simulink model "PMSM_MPCC"  (R2022b)
settings: Solver=FixedStepDiscrete  StartTime=0.0  StopTime=0.5  FixedStep=1e-6  RelTol=1e-3
model workspace (MAT data in the model file):
  B = 0
  Current_Filter_On = 0
  F = 10000
  J = 5.8e-05
  Ls = 0.0005125
  Pn = 5
  Rs = 0.1445
  T = 0.0001
  T_deadband = 3e-06
  Ts = 5e-05
  Vdc = 60
  psi_f = 0.0113
  speed_ki = 1.2
  speed_kp = 0.7
undefined symbols (not defined in the file): sigbuilder_block
libraries: spsDCVoltageSourceLib x1, dspstat3 x1, spsPermanentMagnetSynchronousMachineLib x1, slpidlib x1, spsTwoLevelConverterLib x1, spspowerguiLib x1, simulink x1
(part 1 of 2)
settings Model: Creator=A  LastModifiedBy=31904
settings ModelReferenceCC: EnableRefExpFcnMdlSchedulingChecks=on

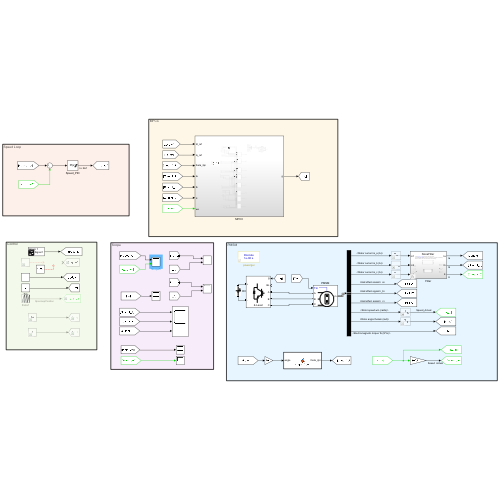
[thumbnail: Simulink's stored preview of the top-level diagram]
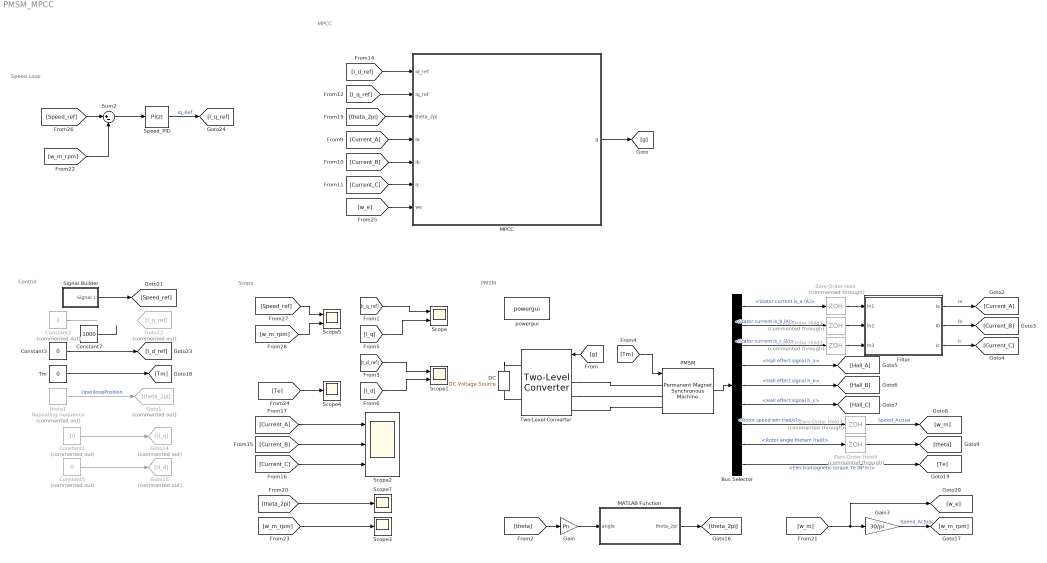
== system PMSM_MPCC ==
  note: Speed Loop
  note: Scope
  note: Control
  note: MPCC
  note: PMSM
  Bus Selector : BusSelector  OutputSignals=Stator current is_a (A),Stator current is_b (A),Stator current is_c (A),Hall effect signal h_a,Hall effect signal h_b,Hall effect signal h_c,Rotor speed wm (rad/s),Rotor angle thetam (rad),Electromagnetic torque Te (N*m)
  Constant1 : Constant  Commented=on  Value=10
  Constant2 : Constant  Commented=on  Value=2
  Constant3 : Constant  Value=0
  Constant5 : Constant  Commented=on  Value=0
  Constant7 : Constant  Value=1000
  DC : spsDCVoltageSourceLib/DC Voltage Source  Amplitude=Vdc  Measurements=None
  Filter : Subsystem  Variant=on
  Gain : Gain  Gain=Pn
  Gain3 : Gain  Gain=30/pi
  Goto1 : Goto  Commented=on  GotoTag=theta_2pi
  Goto14 : Goto  Commented=on  GotoTag=U_q
  Goto15 : Goto  Commented=on  GotoTag=U_d
  Goto22 : Goto  Commented=on  GotoTag=I_q_ref
  MATLAB Function : MATLAB Function  TreatAsAtomicUnit=on
  MPCC : Subsystem
  PMSM : spsPermanentMagnetSynchronousMachineLib/Permanent Magnet Synchronous Machine  NbPhases=3  FluxDistribution=Sinusoidal  RotorType=Round  MechanicalLoad=Torque Tm  PresetModel=No  ShowDetailedParameters=on  MeasurementBus=off  Resistance=Rs  Inductance=8.5e-3  dqInductances=[8.5e-3,8.5e-3]  La=Ls  MachineConstant=Flux linkage established by magnets (V.s)  Flux=psi_f  VoltageCst=10.248  TorqueCst=0.08475  Flat=120  Mechanical=[J B Pn 0]  PolePairs=4  InitialConditions=[0,0, 0,0]  InitialConditions5ph=[0 0 0 0 0 0]  RefAngle=Aligned with phase A axis (original Park)  IterativeDiscreteModel=Trapezoidal non iterative  TsBlock=-1  TsPowergui=0
  Scope : Scope  NumInputPorts=2
  Scope1 : Scope  NumInputPorts=2
  Scope2 : Scope  NumInputPorts=3
  Scope3 : Scope
  Scope4 : Scope
  Scope5 : Scope  NumInputPorts=2
  Scope7 : Scope
  Signal Builder : Subsystem  Tag=STV Subsys  LoadFcn=sigbuilder_block('load');  StartFcn=sigbuilder_block('start');  StopFcn=sigbuilder_block('stop');  ClipboardFcn=sigbuilder_block('clipboard');  mask(Sigbuilder block){tuvar=[0:10]}
      mask help: Simulink:masks:SigbuilderBlock_MD
      mask init:
      | if ~strcmp(get_param(bdroot(gcbh),'SimulationStatus'),'stopped') tuvar = sigbuilder_block('maskInit'); end
      settings: CopyFcn=sigbuilder_block('copy');  DeleteFcn=sigbuilder_block('delete');  ModelCloseFcn=sigbuilder_block('modelClose');  PreSaveFcn=sigbuilder_block('preSave');  PauseFcn=sigbuilder_block('pause');  ContinueFcn=sigbuilder_block('continue');  NameChangeFcn=sigbuilder_block('namechange');  OpenFcn=sigbuilder_block('open',[0 0 1152 596.4 ]);  CloseFcn=sigbuilder_block('close');
      mask Display: plot(0, 0, 100, 100,[2, 2, 32, 32, 2], [68, 8, 8, 68, 68],[32, 2], [38, 38], [32, 19, 2],[53, 60, 44], [32, 17, 17, 2],[16, 16, 31, 31]);txt = getActiveGroup(gcbh);text(2, 100, txt,'verticalAlignment', 'top');
  Speed_PID : slpidlib/PID Controller  Controller=PI  Form=Parallel  TimeDomain=Discrete-time  UseExternalTs=off  SampleTime=-1  IntegratorMethod=Forward Euler  FilterMethod=Forward Euler  ControllerParametersSource=internal  P=speed_kp  I=speed_ki  UseKiTs=off  D=0  N=100  UseFilter=on  TunerSelectOption=Transfer Function Based (PID Tuner App)  InitialConditionSource=internal  InitialConditionForIntegrator=0  InitialConditionForFilter=0  DifferentiatorICPrevScaledInput=0  ExternalReset=none  TrackingMode=off  Kt=1  LimitOutput=on  SatLimitsSource=internal  UpperSaturationLimit=Vdc  LowerSaturationLimit=-Vdc  LinearizeAsGain=on  AntiWindupMode=back-calculation  Kb=0.5  LimitIntegrator=off  UpperIntegratorSaturationLimit=inf  LowerIntegratorSaturationLimit=-inf  POutMin=[]  POutMax=[]  IOutMin=[]  IOutMax=[]  DOutMin=[]  DOutMax=[]  NOutMin=[]  NOutMax=[]  SumOutMin=[]  SumOutMax=[]  SaturationOutMin=[]  SaturationOutMax=[]  PParamMin=[]  PParamMax=[]  IParamMin=[]  IParamMax=[]  DParamMin=[]  DParamMax=[]  NParamMin=[]  NParamMax=[]  KbParamMin=[]  KbParamMax=[]  KtParamMin=[]  KtParamMax=[]  KbOutMin=[]  KbOutMax=[]  KtOutMin=[]  KtOutMax=[]  IntegratorOutMin=[]  IntegratorOutMax=[]  FilterOutMin=[]  FilterOutMax=[]  SumI1OutMin=[]  SumI1OutMax=[]  SumI2OutMin=[]  SumI2OutMax=[]  SumI3OutMin=[]  SumI3OutMax=[]  SumI4OutMin=[]  SumI4OutMax=[]  SumDOutMin=[]  SumDOutMax=[]  DifferentiatorOutMin=[]  DifferentiatorOutMax=[]  FilterDiffOutCoefMin=[]  FilterDiffOutCoefMax=[]  ReciprocalOutMin=[]  ReciprocalOutMax=[]  SumDenOutMin=[]  SumDenOutMax=[]  SumNumOutMin=[]  SumNumOutMax=[]  DivideOutMin=[]  DivideOutMax=[]  UdiffTsProdOutMin=[]  UdiffTsProdOutMax=[]  NTsProdOutMin=[]  NTsProdOutMax=[]  UintegralTsProdOutMin=[]  UintegralTsProdOutMax=[]  UngainTsProdOutMin=[]  UngainTsProdOutMax=[]  ClampingZeroOutDataTypeStr=Inherit: Inherit via back propagation  ClampingZeroOutMin=[]  ClampingZeroOutMax=[]  FilterDenConstantOutDataTypeStr=Inherit: Inherit via back propagation  FilterDenConstantOutMin=[]  FilterDenConstantOutMax=[]  PCopyOutDataTypeStr=Inherit: Inherit via back propagation  PCopyOutMin=[]  PCopyOutMax=[]  NCopyOutDataTypeStr=Inherit: Inherit via back propagation  NCopyOutMin=[]  NCopyOutMax=[]  IntegratorContinuousStateAttributes=''  IntegratorStateMustResolveToSignalObject=off  IntegratorRTWStateStorageClass=Auto  FilterContinuousStateAttributes=''  FilterStateMustResolveToSignalObject=off  FilterRTWStateStorageClass=Auto  ParallelPVariant=InternalParameters  IdealPVariant=Disabled  IVariant=InternalParameters  DVariant=Disabled  IntegratorVariant=Discrete  SatVariant=Enabled  AWVariant=BackCalculation  PCopyVariant=Disabled  TRVariant=Disabled  FdbkBlocksVariant=Forward  IdealPFdbkVariant=Disabled  SatFdbkVariant=Disabled  DerivativeFilterVariant=Disabled  NVariant=Disabled  NCopyVariant=Disabled_SignalSpec  FilterICVariant=Disabled  IntegratorICVariant=InternalICs  ExternalResetVariant=Disabled  TRSumVariant=Passthrough  SumFdbkVariant=Disabled  SumVariant=Sum_PI  TsampFilterVariant=InternalTs  TsampNgainVariant=Passthrough  TsampIntegralVariant=Passthrough  ExternalSaturationOutDataTypeStr=Inherit: Same as second input
  Sum2 : Sum  Inputs=|+-
  Tm : Constant  Value=0
  Two-Level Converter : spsTwoLevelConverterLib/Two-Level Converter  ModelType=Switching devices  Ron=1e-3  Rs=1e6  Cs=inf  Vforward=[0,0]  Ron_Diode=1e-3  Rs_Diode=1e6  Cs_Diode=inf  Vf_Diode=1e-3  Rs_CurrentSource=inf  Ron_ACsource=1e-3
  Zero-Order Hold{,1..4} (5 alike) : ZeroOrderHold  Commented=through  SampleTime=1/F
  powergui : spspowerguiLib/powergui  Priority=1  SimulationMode=Discrete  SampleTime=1e-6  frequency=60  Iterations=50  frequencyindice=0  Pbase=100e6  ErrMax=1e-4  UnitsV=kV  UnitsW=MW  buscounter=0  FunctionMessages=off  echomessages=off  EnableUseOfTLC=off  CurrentSourceSwitches=off  DisableSnubberDevices=off  DisableRonSwitches=off  DisableVfSwitches=off  DisplayEquations=off  AutomaticDiscreteSolvers=off  SolverType=Tustin/Backward Euler (TBE)  Interpol=off  ExternalGateDelay=off  methode=off  Ts=100  x0status=blocks  SPID=on  SwTol=0  HookPort=off  NonlinearTolerance=1e-4  nMaxIteration=100  ContinueOnMaxIteration=off  RestoreLinks=warning  ResistiveCurrentMeasurement=off  Frange=[0:2:500]  Ylog=off  Xlog=on  ShowGrid=off  save=off  variable=ZData  structure=0  ZoomFFT=off  StartTime=0.0  cycles=1  DisplayStyle=1  fundamental=60  FreqAxis=off  MaxFrequency=1000  frequencyindicesteady=1  RmsSteady=1  display=off
  theta1 : simulink/Sources/Repeating Sequence  Commented=on  rep_seq_t=[0 0.1]  rep_seq_y=[0 2*pi]
  wires:
  [theta_2pi] -> MPCC/3(theta_2pi)
  [Current_A] -> MPCC/4(Ia)
  [Current_C] -> MPCC/6(Ic)
  [Current_B] -> MPCC/5(Ib)
  Zero-Order Hold4/1 -> [theta]
  Bus Selector/1 -> Zero-Order Hold/1  "<Stator current is_a (A)>"
  Zero-Order Hold/1 -> Filter/1(ln1)
  Zero-Order Hold1/1 -> Filter/2(ln2)
  Bus Selector/4 -> [Hall_A]  "<Hall effect signal h_a>"
  [theta] -> Gain/1
  Bus Selector/2 -> Zero-Order Hold1/1  "<Stator current is_b (A)>"
  [g] -> Two-Level Converter/1
  Bus Selector/3 -> Zero-Order Hold2/1  "<Stator current is_c (A)>"
  [Tm] -> PMSM/1
  Zero-Order Hold3/1 -> [w_m]  "Speed_Actual"
  Bus Selector/8 -> Zero-Order Hold4/1  "<Rotor angle thetam (rad)>"
  MATLAB Function/1(theta_2pi) -> [theta_2pi]
  Bus Selector/7 -> Zero-Order Hold3/1  "<Rotor speed wm (rad/s)>"
  PMSM/1 -> Bus Selector/1
  Bus Selector/5 -> [Hall_B]  "<Hall effect signal h_b>"
  Zero-Order Hold2/1 -> Filter/3(ln3)
  Bus Selector/6 -> [Hall_C]  "<Hall effect signal h_c>"
  Constant3/1 -> [I_d_ref]
  Constant2/1 -> ?
  [I_q_ref] -> Scope/1
  [I_q] -> Scope/2
  [I_d_ref] -> Scope1/1
  [I_d] -> Scope1/2
  [I_q_ref] -> MPCC/2(Iq_ref)
  [Current_C] -> Scope2/3
  [Current_B] -> Scope2/2
  [Current_A] -> Scope2/1
  [theta_2pi] -> Scope7/1
  Filter/1(Ia) -> [Current_A]  "Ia"
  Filter/2(Ib) -> [Current_B]  "Ib"
  Filter/3(Ic) -> [Current_C]  "Ic"
  MPCC/1(g) -> [g]
  theta1/1 -> Goto1/1  "OpenloopPosition"
  Constant5/1 -> Goto15/1
  Constant1/1 -> Goto14/1
  [w_m] -> [w_e], Gain3/1
  Gain3/1 -> [w_m_rpm]  "Speed_Actual"
  [w_m_rpm] -> Scope3/1
  Gain/1 -> MATLAB Function/1(angle)
  Tm/1 -> [Tm]
  Bus Selector/9 -> [Te]  "<Electromagnetic torque Te (N*m)>"
  [Te] -> Scope4/1
  [w_e] -> MPCC/7(we)
  Constant7/1 -> ?
  Sum2/1 -> Speed_PID/1
  [w_m_rpm] -> Sum2/2
  [Speed_ref] -> Sum2/1
  Speed_PID/1 -> [I_q_ref]  "Iq_Ref"
  [Speed_ref] -> Scope5/1
  [w_m_rpm] -> Scope5/2
  Signal Builder/1(Signal 1) -> [Speed_ref]
  [I_d_ref] -> MPCC/1(Id_ref)
  connections:
  DC/LConn1 -- Two-Level Converter/RConn2
  DC/RConn1 -- Two-Level Converter/RConn1
  PMSM/LConn3 -- Two-Level Converter/LConn3
  Two-Level Converter/LConn1 -- PMSM/LConn1
  Two-Level Converter/LConn2 -- PMSM/LConn2

== system PMSM_MPCC/Filter ==
  note: 1) Add Subsystem or Model blocks as valid variant choices.
      | 2) You cannot connect blocks at this level. At simulation, connectivity is automatically
      | determined, based on the active variant and port name matching.
  ln1 : Inport
  ln2 : Inport  Port=2
  ln3 : Inport  Port=3
  LowpassFilter : Subsystem  VariantControl=Current_Filter_On==1
  NoneFilter : Subsystem  VariantControl=Current_Filter_On==0
  Ia : Outport
  Ib : Outport  Port=2
  Ic : Outport  Port=3

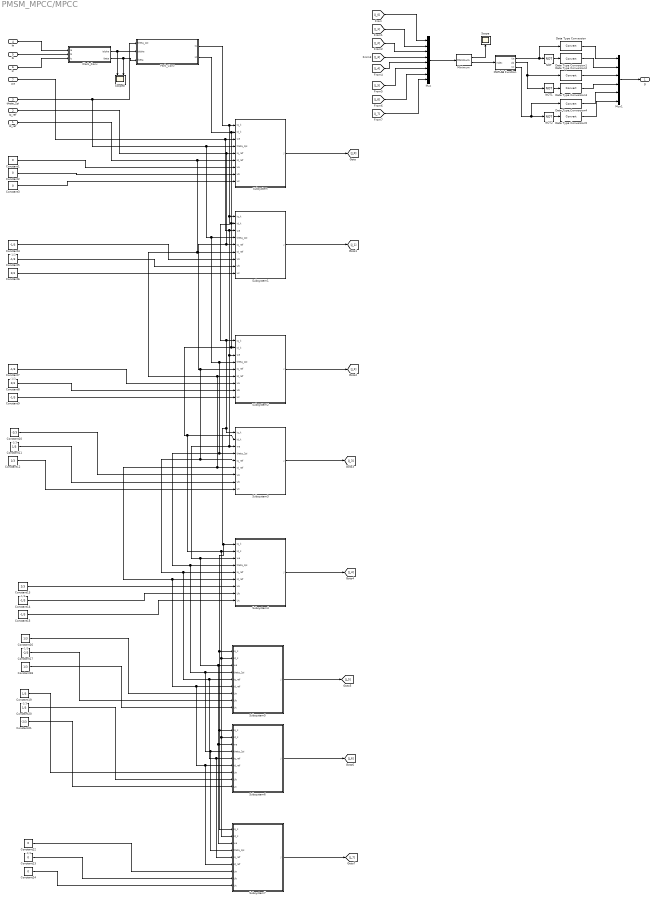
== system PMSM_MPCC/MPCC ==
  note: -1/3
  note: -1/3
  note: -1/3
  note: -1/3
  note: -1/3
  note: -1/3
  note: -1/3
  Id_ref : Inport
  Iq_ref : Inport  Port=2
  theta_2pi : Inport  Port=3
  Ia : Inport  Port=4
  Ib : Inport  Port=5
  Ic : Inport  Port=6
  we : Inport  Port=7
  Clark_Conv : Subsystem
  Constant{1..3,22..24} (6 alike) : Constant  Value=0
  Constant10 : Constant  Value=-2/3
  Constant{11..12,16,18..20} (6 alike) : Constant  Value=1/3
  Constant13 : Constant  Value=2/3
  Constant{4..5,7,9,14..15} (6 alike) : Constant  Value=-1/3
  Constant17 : Constant  Value=-2/3
  Constant21 : Constant  Value=-2/3
  Constant6 : Constant  Value=2/3
  Constant8 : Constant  Value=2/3
  Data Type Conversion{,1..5} (6 alike) : DataTypeConversion  SaturateOnIntegerOverflow=off  RndMeth=Floor
  MATLAB Function : MATLAB Function  TreatAsAtomicUnit=on
  Minimum : dspstat3/Minimum  operation=minimum  fcn=Value and Index  indexBase=Zero  operateOver=Entire input  Dimension=1  InputProcessing=Columns as channels (frame based)  reset=None  roiEnable=off  roiType=Rectangles  roiPortion=Entire ROI  roiOutput=Individual statistics for each ROI  roiFlag=off  roundingMode=Floor  overflowMode=off
      settings: LibrarySourceBlock=dsphdlsupportstat/Minimum
  Mux : Mux  Inputs=8
  Mux1 : Mux  Inputs=6
  NOT : Logic  Operator=NOT  IconShape=distinctive  AllPortsSameDT=off  OutDataTypeStr=boolean
  NOT1 : Logic  Operator=NOT  IconShape=distinctive  AllPortsSameDT=off  OutDataTypeStr=boolean
  NOT2 : Logic  Operator=NOT  IconShape=distinctive  AllPortsSameDT=off  OutDataTypeStr=boolean
  Park_Conv : Subsystem
  Scope : Scope
  Scope8 : Scope  NumInputPorts=2
  Subsystem : Subsystem
  Subsystem1 : Subsystem
  Subsystem2 : Subsystem
  Subsystem3 : Subsystem
  Subsystem4 : Subsystem
  Subsystem5 : Subsystem
  Subsystem6 : Subsystem
  Subsystem7 : Subsystem
  g : Outport
  wires:
  Clark_Conv/1(Ialpha) -> Park_Conv/2(Ialpha), Scope8/1
  theta_2pi/1 -> Park_Conv/1(theta_2pi), Subsystem/4(theta_2pi), Subsystem3/4(theta_2pi), Subsystem7/4(theta_2pi), Subsystem6/4(theta_2pi), Subsystem5/4(theta_2pi), Subsystem4/4(theta_2pi), Subsystem2/4(theta_2pi), Subsystem1/4(theta_2pi)
  Clark_Conv/2(Ibeta) -> Park_Conv/3(Ibeta), Scope8/2
  Mux1/1 -> g/1
  Ic/1 -> Clark_Conv/3(Ic)
  Ib/1 -> Clark_Conv/2(Ib)
  Ia/1 -> Clark_Conv/1(Ia)
  Constant22/1 -> Subsystem7/7(Ua)
  Constant24/1 -> Subsystem7/9(Uc)
  Constant12/1 -> Subsystem3/9(Uc)
  Constant19/1 -> Subsystem6/7(Ua)
  Constant20/1 -> Subsystem6/8(Ub)
  Constant11/1 -> Subsystem3/8(Ub)
  Constant10/1 -> Subsystem3/7(Ua)
  Constant7/1 -> Subsystem2/7(Ua)
  Constant8/1 -> Subsystem2/8(Ub)
  Constant9/1 -> Subsystem2/9(Uc)
  Constant4/1 -> Subsystem1/7(Ua)
  Constant5/1 -> Subsystem1/8(Ub)
  Constant6/1 -> Subsystem1/9(Uc)
  Constant17/1 -> Subsystem5/8(Ub)
  Constant23/1 -> Subsystem7/8(Ub)
  Constant16/1 -> Subsystem5/7(Ua)
  Constant15/1 -> Subsystem4/9(Uc)
  Constant18/1 -> Subsystem5/9(Uc)
  Constant21/1 -> Subsystem6/9(Uc)
  Constant14/1 -> Subsystem4/8(Ub)
  Constant13/1 -> Subsystem4/7(Ua)
  Park_Conv/1(Iq) -> Subsystem7/1(iq_k), Subsystem6/1(iq_k), Subsystem5/1(iq_k), Subsystem4/1(iq_k), Subsystem3/1(iq_k), Subsystem2/1(iq_k), Subsystem1/1(iq_k), Subsystem/1(iq_k)
  Park_Conv/2(Id) -> Subsystem7/2(id_k), Subsystem6/2(id_k), Subsystem5/2(id_k), Subsystem4/2(id_k), Subsystem3/2(id_k), Subsystem2/2(id_k), Subsystem1/2(id_k), Subsystem/2(id_k)
  we/1 -> Subsystem3/3(we), Subsystem7/3(we), Subsystem6/3(we), Subsystem5/3(we), Subsystem4/3(we), Subsystem2/3(we), Subsystem1/3(we), Subsystem/3(we)
  Iq_ref/1 -> Subsystem1/5(Iq_ref), Subsystem3/5(Iq_ref), Subsystem7/5(Iq_ref), Subsystem6/5(Iq_ref), Subsystem5/5(Iq_ref), Subsystem4/5(Iq_ref), Subsystem2/5(Iq_ref), Subsystem/5(Iq_ref)
  Id_ref/1 -> Subsystem1/6(Id_ref), Subsystem3/6(Id_ref), Subsystem7/6(Id_ref), Subsystem6/6(Id_ref), Subsystem5/6(Id_ref), Subsystem4/6(Id_ref), Subsystem2/6(Id_ref), Subsystem/6(Id_ref)
  Constant1/1 -> Subsystem/7(Ua)
  Constant2/1 -> Subsystem/8(Ub)
  Constant3/1 -> Subsystem/9(Uc)
  Subsystem/1(J) -> [J_0]
  Subsystem1/1(J) -> [J_1]
  Subsystem2/1(J) -> [J_2]
  Subsystem3/1(J) -> [J_3]
  Subsystem4/1(J) -> [J_4]
  Subsystem5/1(J) -> [J_5]
  Subsystem6/1(J) -> [J_6]
  Subsystem7/1(J) -> [J_7]
  [J_0] -> Mux/1
  [J_1] -> Mux/2
  [J_2] -> Mux/3
  [J_3] -> Mux/4
  [J_4] -> Mux/5
  [J_5] -> Mux/6
  [J_6] -> Mux/7
  [J_7] -> Mux/8
  Mux/1 -> Minimum/1
  Minimum/1 -> Scope/1
  Minimum/2 -> MATLAB Function/1(index)
  MATLAB Function/1(Ua) -> Data Type Conversion/1, NOT/1
  NOT/1 -> Data Type Conversion1/1
  Data Type Conversion/1 -> Mux1/1
  Data Type Conversion1/1 -> Mux1/2
  Data Type Conversion2/1 -> Mux1/3
  Data Type Conversion3/1 -> Mux1/4
  NOT1/1 -> Data Type Conversion3/1
  MATLAB Function/2(Ub) -> Data Type Conversion2/1, NOT1/1
  Data Type Conversion4/1 -> Mux1/5
  Data Type Conversion5/1 -> Mux1/6
  NOT2/1 -> Data Type Conversion5/1
  MATLAB Function/3(Uc) -> Data Type Conversion4/1, NOT2/1

== system PMSM_MPCC/Signal Builder ==
  Demux : Demux  Tag=STV Demux  Outputs=1
      settings: DisplayOption=none
  FromWs : FromWorkspace  Tag=STV FromWs  VariableName=tuvar
      SigBuilderData=|
      | common.afterFinalStr = 'Extrapolate'
      | common.sampleTime = 0
      | dataSet.timeRange = [0 1]
      | dataSet.name = 'Group 1'
      | sbobj.Groups.Name = 'Group 1'
      | sbobj.Groups.Signals.Name = 'Signal 1'
      | sbobj.Groups.Signals.XData = [0 0.2 0.2 0.3 0.3 0.5 0.5 0.6 0.6 0.8 0.8 0.9 0.9 1]
      | sbobj.Groups.Signals.YData = [1000 1000 3000 3000 5000 5000 4000 4000 2000 2000 1000 1000 0 0]
      | sbobj.Groups.TimeRange = [0 1]
  Signal 1 : Outport  Tag=STV Outport
  wires:
  Demux/1 -> Signal 1/1
  FromWs/1 -> Demux/1

== system PMSM_MPCC/Filter/LowpassFilter ==
  ln1 : Inport
  ln2 : Inport  Port=2
  ln3 : Inport  Port=3
  Lowpass filter1 : Subsystem
  Lowpass filter2 : Subsystem
  Lowpass filter3 : Subsystem
  a : Constant  Value=0.001
  Ia : Outport
  Ib : Outport  Port=2
  Ic : Outport  Port=3
  wires:
  ln2/1 -> Lowpass filter2/2(u(t))
  a/1 -> Lowpass filter3/1(K), Lowpass filter2/1(K), Lowpass filter1/1(K)
  ln1/1 -> Lowpass filter1/2(u(t))
  Lowpass filter1/1(Ia) -> Ia/1
  Lowpass filter2/1(Ib) -> Ib/1
  Lowpass filter3/1(Ic) -> Ic/1
  ln3/1 -> Lowpass filter3/2(u(t))

== system PMSM_MPCC/Filter/NoneFilter ==
  ln1 : Inport
  ln2 : Inport  Port=2
  ln3 : Inport  Port=3
  Ia : Outport
  Ib : Outport  Port=2
  Ic : Outport  Port=3
  wires:
  ln1/1 -> Ia/1
  ln2/1 -> Ib/1
  ln3/1 -> Ic/1

== system PMSM_MPCC/MPCC/Clark_Conv ==
  Ia : Inport
  Ib : Inport  Port=2
  Ic : Inport  Port=3
  Add : Sum  Inputs=+-  OutDataTypeStr=double
  Gain : Gain  Gain=sqrt(3)  ParamDataTypeStr=double
  Gain2 : Gain  Gain=0.5
  Gain3 : Gain  Gain=0.5
  Subtract : Sum  Inputs=+--  OutDataTypeStr=double
  Ialpha : Outport
  Ibeta : Outport  Port=2
  wires:
  Ia/1 -> Subtract/1
  Ib/1 -> Gain2/1
  Add/1 -> Gain/1
  Gain/1 -> Ibeta/1
  Ic/1 -> Gain3/1
  Gain2/1 -> Subtract/2, Add/1
  Gain3/1 -> Subtract/3, Add/2
  Subtract/1 -> Ialpha/1

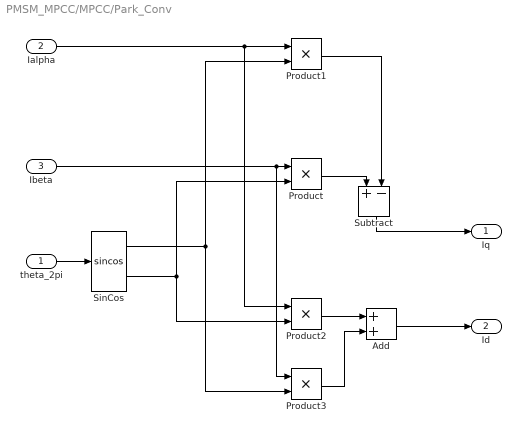
== system PMSM_MPCC/MPCC/Park_Conv ==
  theta_2pi : Inport
  Ialpha : Inport  Port=2
  Ibeta : Inport  Port=3
  Add : Sum
  Product{,1..3} (4 alike) : Product
  SinCos : Trigonometry  Operator=sincos
  Subtract : Sum  Inputs=+-
  Iq : Outport
  Id : Outport  Port=2
  wires:
  Ialpha/1 -> Product1/1, Product2/1
  Ibeta/1 -> Product3/1, Product/1
  theta_2pi/1 -> SinCos/1
  SinCos/2 -> Product2/2, Product/2
  SinCos/1 -> Product3/2, Product1/2
  Product1/1 -> Subtract/2
  Subtract/1 -> Iq/1
  Product/1 -> Subtract/1
  Product2/1 -> Add/1
  Product3/1 -> Add/2
  Add/1 -> Id/1

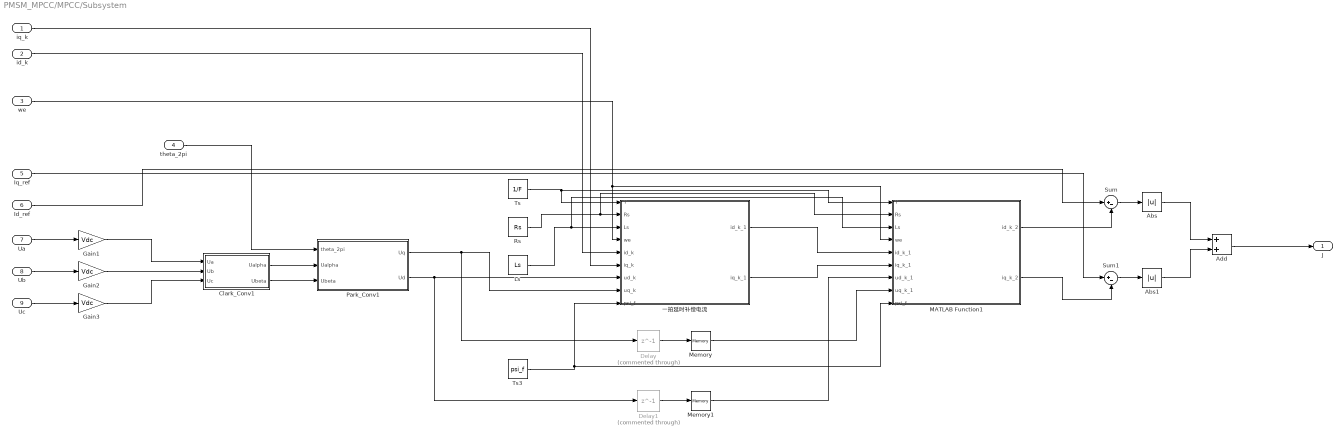
== system PMSM_MPCC/MPCC/Subsystem ==
  iq_k : Inport
  id_k : Inport  Port=2
  we : Inport  Port=3
  theta_2pi : Inport  Port=4
  Iq_ref : Inport  Port=5
  Id_ref : Inport  Port=6
  Ua : Inport  Port=7
  Ub : Inport  Port=8
  Uc : Inport  Port=9
  Abs : Abs  SaturateOnIntegerOverflow=off
  Abs1 : Abs  SaturateOnIntegerOverflow=off
  Add : Sum
  Clark_Conv1 : Subsystem
  Delay : Delay  Commented=through  DelayLength=1
  Delay1 : Delay  Commented=through  DelayLength=1
  Gain1 : Gain  Gain=Vdc
  Gain2 : Gain  Gain=Vdc
  Gain3 : Gain  Gain=Vdc
  Ls : Constant  Value=Ls
  MATLAB Function1 : MATLAB Function  TreatAsAtomicUnit=on
  Memory : Memory
  Memory1 : Memory
  Park_Conv1 : Subsystem
  Rs : Constant  Value=Rs
  Sum : Sum  Inputs=|+-
  Sum1 : Sum  Inputs=|+-
  Ts : Constant  Value=1/F
  Ts3 : Constant  Value=psi_f
  一拍延时补偿电流 : MATLAB Function  TreatAsAtomicUnit=on
  J : Outport
  wires:
  Park_Conv1/1(Uq) -> Delay/1, 一拍延时补偿电流/8(uq_k)
  MATLAB Function1/2(iq_k_2) -> Sum1/2
  Iq_ref/1 -> Sum1/1
  theta_2pi/1 -> Park_Conv1/1(theta_2pi)
  Sum/1 -> Abs/1
  一拍延时补偿电流/2(iq_k_1) -> MATLAB Function1/6(iq_k_1)
  Rs/1 -> MATLAB Function1/2(Rs), 一拍延时补偿电流/2(Rs)
  Delay/1 -> Memory/1
  MATLAB Function1/1(id_k_2) -> Sum/2
  Add/1 -> J/1
  Ts/1 -> MATLAB Function1/1(T), 一拍延时补偿电流/1(T)
  一拍延时补偿电流/1(id_k_1) -> MATLAB Function1/5(id_k_1)
  Park_Conv1/2(Ud) -> Delay1/1, 一拍延时补偿电流/7(ud_k)
  Gain1/1 -> Clark_Conv1/1(Ua)
  Gain2/1 -> Clark_Conv1/2(Ub)
  Ls/1 -> MATLAB Function1/3(Ls), 一拍延时补偿电流/3(Ls)
  Clark_Conv1/2(Ubeta) -> Park_Conv1/3(Ubeta)
  Sum1/1 -> Abs1/1
  Gain3/1 -> Clark_Conv1/3(Uc)
  Abs/1 -> Add/1
  Id_ref/1 -> Sum/1
  we/1 -> 一拍延时补偿电流/4(we), MATLAB Function1/4(we)
  Delay1/1 -> Memory1/1
  Ua/1 -> Gain1/1
  Ts3/1 -> MATLAB Function1/9(psi_f), 一拍延时补偿电流/9(psi_f)
  Abs1/1 -> Add/2
  Clark_Conv1/1(Ualpha) -> Park_Conv1/2(Ualpha)
  id_k/1 -> 一拍延时补偿电流/5(id_k)
  iq_k/1 -> 一拍延时补偿电流/6(iq_k)
  Ub/1 -> Gain2/1
  Uc/1 -> Gain3/1
  Memory/1 -> MATLAB Function1/8(uq_k_1)
  Memory1/1 -> MATLAB Function1/7(ud_k_1)

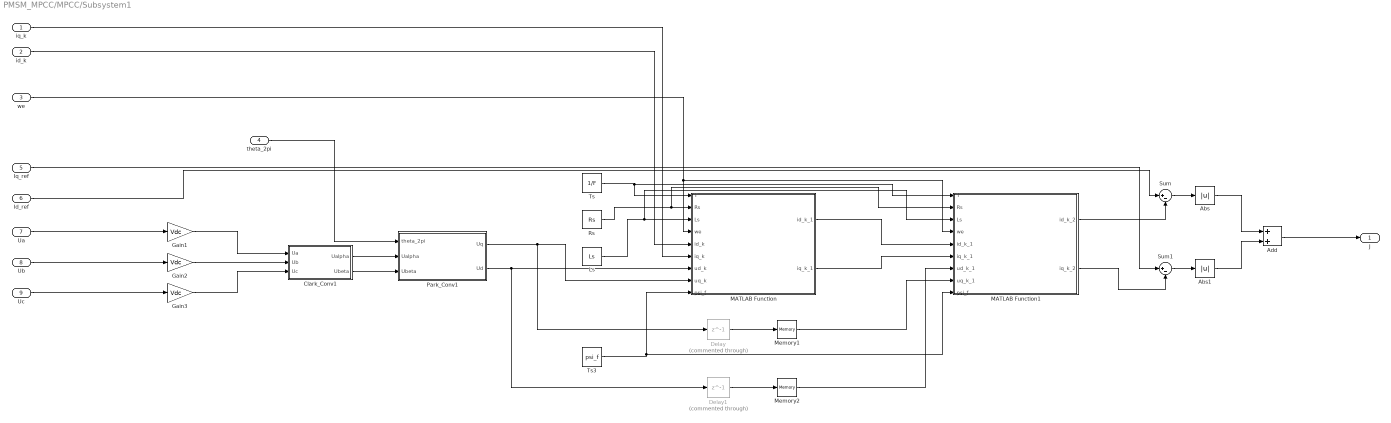
== system PMSM_MPCC/MPCC/Subsystem1 ==
  iq_k : Inport
  id_k : Inport  Port=2
  we : Inport  Port=3
  theta_2pi : Inport  Port=4
  Iq_ref : Inport  Port=5
  Id_ref : Inport  Port=6
  Ua : Inport  Port=7
  Ub : Inport  Port=8
  Uc : Inport  Port=9
  Abs : Abs  SaturateOnIntegerOverflow=off
  Abs1 : Abs  SaturateOnIntegerOverflow=off
  Add : Sum
  Clark_Conv1 : Subsystem
  Delay : Delay  Commented=through  DelayLength=1
  Delay1 : Delay  Commented=through  DelayLength=1
  Gain1 : Gain  Gain=Vdc
  Gain2 : Gain  Gain=Vdc
  Gain3 : Gain  Gain=Vdc
  Ls : Constant  Value=Ls
  MATLAB Function : MATLAB Function  TreatAsAtomicUnit=on
  MATLAB Function1 : MATLAB Function  TreatAsAtomicUnit=on
  Memory1 : Memory
  Memory2 : Memory
  Park_Conv1 : Subsystem
  Rs : Constant  Value=Rs
  Sum : Sum  Inputs=|+-
  Sum1 : Sum  Inputs=|+-
  Ts : Constant  Value=1/F
  Ts3 : Constant  Value=psi_f
  J : Outport
  wires:
  Uc/1 -> Gain3/1
  Ub/1 -> Gain2/1
  iq_k/1 -> MATLAB Function/6(iq_k)
  id_k/1 -> MATLAB Function/5(id_k)
  Clark_Conv1/1(Ualpha) -> Park_Conv1/2(Ualpha)
  Abs1/1 -> Add/2
  Ts3/1 -> MATLAB Function/9(psi_f), MATLAB Function1/9(psi_f)
  Ua/1 -> Gain1/1
  Delay1/1 -> Memory2/1
  we/1 -> MATLAB Function1/4(we), MATLAB Function/4(we)
  Id_ref/1 -> Sum/1
  Abs/1 -> Add/1
  Gain3/1 -> Clark_Conv1/3(Uc)
  Sum1/1 -> Abs1/1
  Clark_Conv1/2(Ubeta) -> Park_Conv1/3(Ubeta)
  Ls/1 -> MATLAB Function/3(Ls), MATLAB Function1/3(Ls)
  Gain2/1 -> Clark_Conv1/2(Ub)
  Gain1/1 -> Clark_Conv1/1(Ua)
  Park_Conv1/2(Ud) -> MATLAB Function/7(ud_k), Delay1/1
  MATLAB Function/1(id_k_1) -> MATLAB Function1/5(id_k_1)
  Ts/1 -> MATLAB Function/1(T), MATLAB Function1/1(T)
  Add/1 -> J/1
  MATLAB Function1/1(id_k_2) -> Sum/2
  Delay/1 -> Memory1/1
  Rs/1 -> MATLAB Function/2(Rs), MATLAB Function1/2(Rs)
  MATLAB Function/2(iq_k_1) -> MATLAB Function1/6(iq_k_1)
  Sum/1 -> Abs/1
  theta_2pi/1 -> Park_Conv1/1(theta_2pi)
  Iq_ref/1 -> Sum1/1
  MATLAB Function1/2(iq_k_2) -> Sum1/2
  Park_Conv1/1(Uq) -> MATLAB Function/8(uq_k), Delay/1
  Memory1/1 -> MATLAB Function1/8(uq_k_1)
  Memory2/1 -> MATLAB Function1/7(ud_k_1)

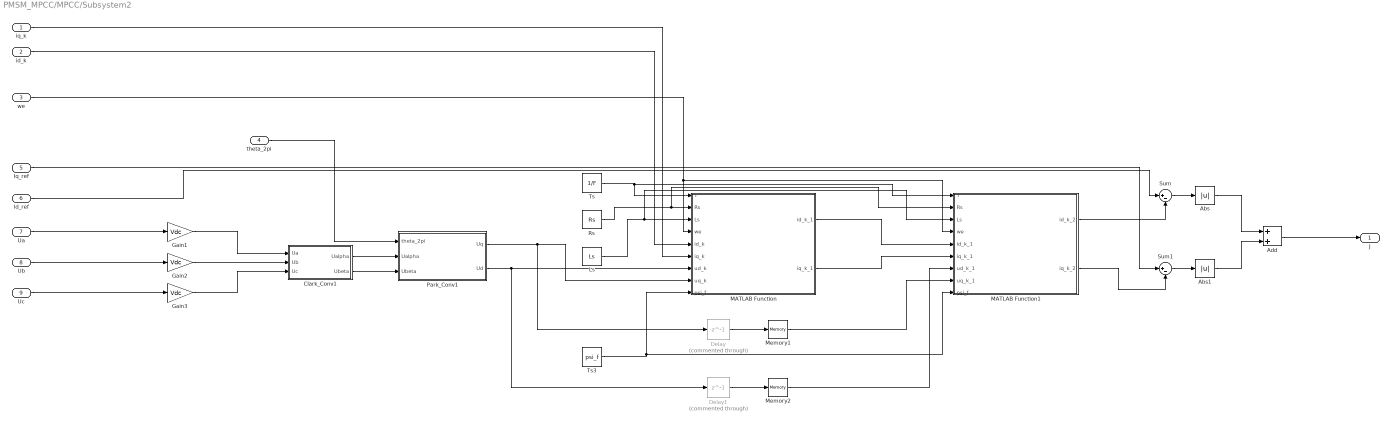
== system PMSM_MPCC/MPCC/Subsystem2 ==
  iq_k : Inport
  id_k : Inport  Port=2
  we : Inport  Port=3
  theta_2pi : Inport  Port=4
  Iq_ref : Inport  Port=5
  Id_ref : Inport  Port=6
  Ua : Inport  Port=7
  Ub : Inport  Port=8
  Uc : Inport  Port=9
  Abs : Abs  SaturateOnIntegerOverflow=off
  Abs1 : Abs  SaturateOnIntegerOverflow=off
  Add : Sum
  Clark_Conv1 : Subsystem
  Delay : Delay  Commented=through  DelayLength=1
  Delay1 : Delay  Commented=through  DelayLength=1
  Gain1 : Gain  Gain=Vdc
  Gain2 : Gain  Gain=Vdc
  Gain3 : Gain  Gain=Vdc
  Ls : Constant  Value=Ls
  MATLAB Function : MATLAB Function  TreatAsAtomicUnit=on
  MATLAB Function1 : MATLAB Function  TreatAsAtomicUnit=on
  Memory1 : Memory
  Memory2 : Memory
  Park_Conv1 : Subsystem
  Rs : Constant  Value=Rs
  Sum : Sum  Inputs=|+-
  Sum1 : Sum  Inputs=|+-
  Ts : Constant  Value=1/F
  Ts3 : Constant  Value=psi_f
  J : Outport
  wires:
  Uc/1 -> Gain3/1
  Ub/1 -> Gain2/1
  iq_k/1 -> MATLAB Function/6(iq_k)
  id_k/1 -> MATLAB Function/5(id_k)
  Clark_Conv1/1(Ualpha) -> Park_Conv1/2(Ualpha)
  Abs1/1 -> Add/2
  Ts3/1 -> MATLAB Function/9(psi_f), MATLAB Function1/9(psi_f)
  Ua/1 -> Gain1/1
  Delay1/1 -> Memory2/1
  we/1 -> MATLAB Function1/4(we), MATLAB Function/4(we)
  Id_ref/1 -> Sum/1
  Abs/1 -> Add/1
  Gain3/1 -> Clark_Conv1/3(Uc)
  Sum1/1 -> Abs1/1
  Clark_Conv1/2(Ubeta) -> Park_Conv1/3(Ubeta)
  Ls/1 -> MATLAB Function/3(Ls), MATLAB Function1/3(Ls)
  Gain2/1 -> Clark_Conv1/2(Ub)
  Gain1/1 -> Clark_Conv1/1(Ua)
  Park_Conv1/2(Ud) -> MATLAB Function/7(ud_k), Delay1/1
  MATLAB Function/1(id_k_1) -> MATLAB Function1/5(id_k_1)
  Ts/1 -> MATLAB Function/1(T), MATLAB Function1/1(T)
  Add/1 -> J/1
  MATLAB Function1/1(id_k_2) -> Sum/2
  Delay/1 -> Memory1/1
  Rs/1 -> MATLAB Function/2(Rs), MATLAB Function1/2(Rs)
  MATLAB Function/2(iq_k_1) -> MATLAB Function1/6(iq_k_1)
  Sum/1 -> Abs/1
  theta_2pi/1 -> Park_Conv1/1(theta_2pi)
  Iq_ref/1 -> Sum1/1
  MATLAB Function1/2(iq_k_2) -> Sum1/2
  Park_Conv1/1(Uq) -> MATLAB Function/8(uq_k), Delay/1
  Memory1/1 -> MATLAB Function1/8(uq_k_1)
  Memory2/1 -> MATLAB Function1/7(ud_k_1)

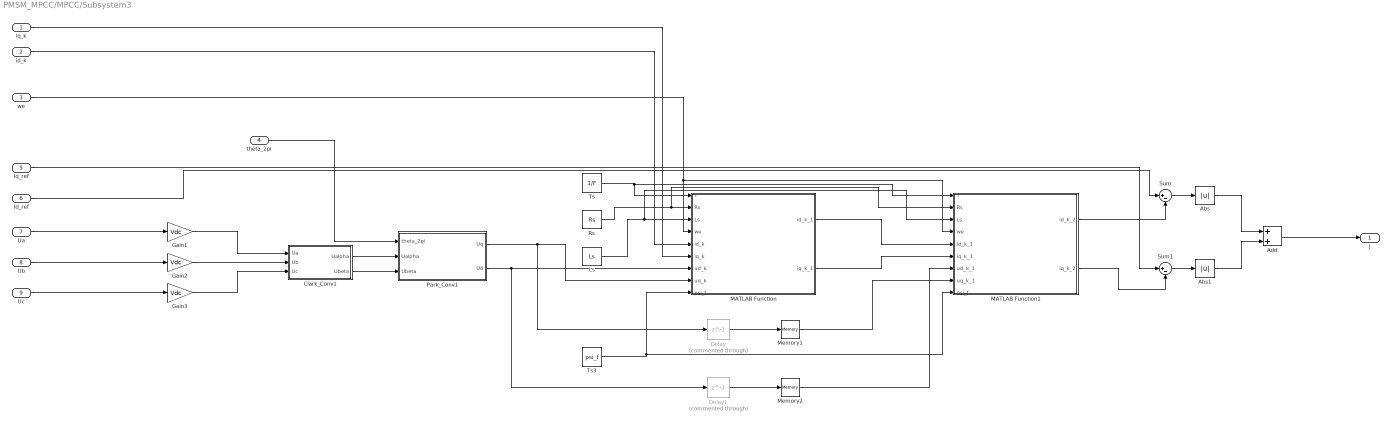
== system PMSM_MPCC/MPCC/Subsystem3 ==
  iq_k : Inport
  id_k : Inport  Port=2
  we : Inport  Port=3
  theta_2pi : Inport  Port=4
  Iq_ref : Inport  Port=5
  Id_ref : Inport  Port=6
  Ua : Inport  Port=7
  Ub : Inport  Port=8
  Uc : Inport  Port=9
  Abs : Abs  SaturateOnIntegerOverflow=off
  Abs1 : Abs  SaturateOnIntegerOverflow=off
  Add : Sum
  Clark_Conv1 : Subsystem
  Delay : Delay  Commented=through  DelayLength=1
  Delay1 : Delay  Commented=through  DelayLength=1
  Gain1 : Gain  Gain=Vdc
  Gain2 : Gain  Gain=Vdc
  Gain3 : Gain  Gain=Vdc
  Ls : Constant  Value=Ls
  MATLAB Function : MATLAB Function  TreatAsAtomicUnit=on
  MATLAB Function1 : MATLAB Function  TreatAsAtomicUnit=on
  Memory1 : Memory
  Memory2 : Memory
  Park_Conv1 : Subsystem
  Rs : Constant  Value=Rs
  Sum : Sum  Inputs=|+-
  Sum1 : Sum  Inputs=|+-
  Ts : Constant  Value=1/F
  Ts3 : Constant  Value=psi_f
  J : Outport
  wires:
  Uc/1 -> Gain3/1
  Ub/1 -> Gain2/1
  iq_k/1 -> MATLAB Function/6(iq_k)
  id_k/1 -> MATLAB Function/5(id_k)
  Clark_Conv1/1(Ualpha) -> Park_Conv1/2(Ualpha)
  Abs1/1 -> Add/2
  Ts3/1 -> MATLAB Function/9(psi_f), MATLAB Function1/9(psi_f)
  Ua/1 -> Gain1/1
  Delay1/1 -> Memory2/1
  we/1 -> MATLAB Function1/4(we), MATLAB Function/4(we)
  Id_ref/1 -> Sum/1
  Abs/1 -> Add/1
  Gain3/1 -> Clark_Conv1/3(Uc)
  Sum1/1 -> Abs1/1
  Clark_Conv1/2(Ubeta) -> Park_Conv1/3(Ubeta)
  Ls/1 -> MATLAB Function/3(Ls), MATLAB Function1/3(Ls)
  Gain2/1 -> Clark_Conv1/2(Ub)
  Gain1/1 -> Clark_Conv1/1(Ua)
  Park_Conv1/2(Ud) -> MATLAB Function/7(ud_k), Delay1/1
  MATLAB Function/1(id_k_1) -> MATLAB Function1/5(id_k_1)
  Ts/1 -> MATLAB Function/1(T), MATLAB Function1/1(T)
  Add/1 -> J/1
  MATLAB Function1/1(id_k_2) -> Sum/2
  Delay/1 -> Memory1/1
  Rs/1 -> MATLAB Function/2(Rs), MATLAB Function1/2(Rs)
  MATLAB Function/2(iq_k_1) -> MATLAB Function1/6(iq_k_1)
  Sum/1 -> Abs/1
  theta_2pi/1 -> Park_Conv1/1(theta_2pi)
  Iq_ref/1 -> Sum1/1
  MATLAB Function1/2(iq_k_2) -> Sum1/2
  Park_Conv1/1(Uq) -> MATLAB Function/8(uq_k), Delay/1
  Memory1/1 -> MATLAB Function1/8(uq_k_1)
  Memory2/1 -> MATLAB Function1/7(ud_k_1)

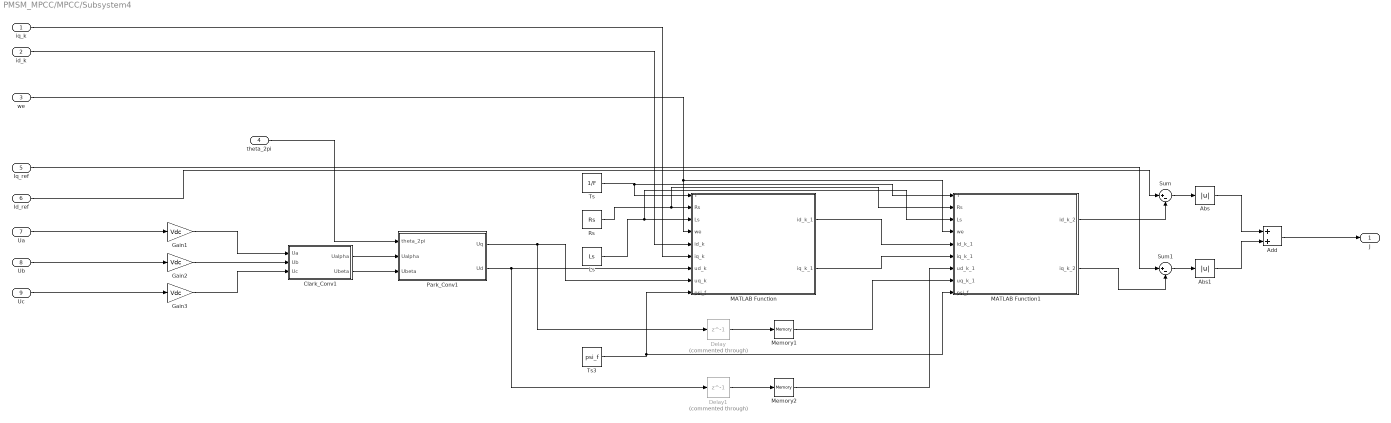
== system PMSM_MPCC/MPCC/Subsystem4 ==
  iq_k : Inport
  id_k : Inport  Port=2
  we : Inport  Port=3
  theta_2pi : Inport  Port=4
  Iq_ref : Inport  Port=5
  Id_ref : Inport  Port=6
  Ua : Inport  Port=7
  Ub : Inport  Port=8
  Uc : Inport  Port=9
  Abs : Abs  SaturateOnIntegerOverflow=off
  Abs1 : Abs  SaturateOnIntegerOverflow=off
  Add : Sum
  Clark_Conv1 : Subsystem
  Delay : Delay  Commented=through  DelayLength=1
  Delay1 : Delay  Commented=through  DelayLength=1
  Gain1 : Gain  Gain=Vdc
  Gain2 : Gain  Gain=Vdc
  Gain3 : Gain  Gain=Vdc
  Ls : Constant  Value=Ls
  MATLAB Function : MATLAB Function  TreatAsAtomicUnit=on
  MATLAB Function1 : MATLAB Function  TreatAsAtomicUnit=on
  Memory1 : Memory
  Memory2 : Memory
  Park_Conv1 : Subsystem
  Rs : Constant  Value=Rs
  Sum : Sum  Inputs=|+-
  Sum1 : Sum  Inputs=|+-
  Ts : Constant  Value=1/F
  Ts3 : Constant  Value=psi_f
  J : Outport
  wires:
  Uc/1 -> Gain3/1
  Ub/1 -> Gain2/1
  iq_k/1 -> MATLAB Function/6(iq_k)
  id_k/1 -> MATLAB Function/5(id_k)
  Clark_Conv1/1(Ualpha) -> Park_Conv1/2(Ualpha)
  Abs1/1 -> Add/2
  Ts3/1 -> MATLAB Function/9(psi_f), MATLAB Function1/9(psi_f)
  Ua/1 -> Gain1/1
  Delay1/1 -> Memory2/1
  we/1 -> MATLAB Function1/4(we), MATLAB Function/4(we)
  Id_ref/1 -> Sum/1
  Abs/1 -> Add/1
  Gain3/1 -> Clark_Conv1/3(Uc)
  Sum1/1 -> Abs1/1
  Clark_Conv1/2(Ubeta) -> Park_Conv1/3(Ubeta)
  Ls/1 -> MATLAB Function/3(Ls), MATLAB Function1/3(Ls)
  Gain2/1 -> Clark_Conv1/2(Ub)
  Gain1/1 -> Clark_Conv1/1(Ua)
  Park_Conv1/2(Ud) -> MATLAB Function/7(ud_k), Delay1/1
  MATLAB Function/1(id_k_1) -> MATLAB Function1/5(id_k_1)
  Ts/1 -> MATLAB Function/1(T), MATLAB Function1/1(T)
  Add/1 -> J/1
  MATLAB Function1/1(id_k_2) -> Sum/2
  Delay/1 -> Memory1/1
  Rs/1 -> MATLAB Function/2(Rs), MATLAB Function1/2(Rs)
  MATLAB Function/2(iq_k_1) -> MATLAB Function1/6(iq_k_1)
  Sum/1 -> Abs/1
  theta_2pi/1 -> Park_Conv1/1(theta_2pi)
  Iq_ref/1 -> Sum1/1
  MATLAB Function1/2(iq_k_2) -> Sum1/2
  Park_Conv1/1(Uq) -> MATLAB Function/8(uq_k), Delay/1
  Memory1/1 -> MATLAB Function1/8(uq_k_1)
  Memory2/1 -> MATLAB Function1/7(ud_k_1)

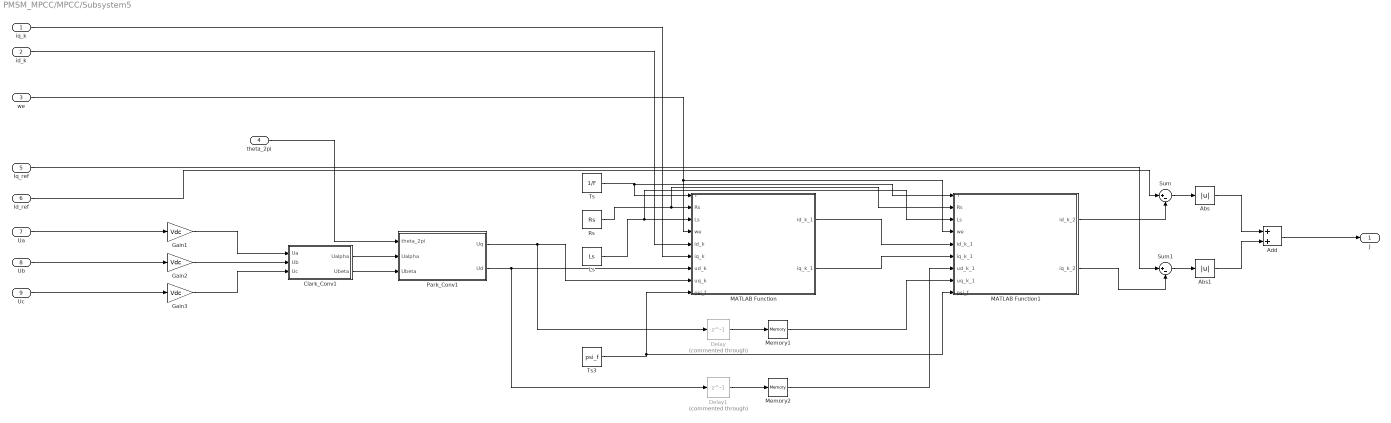
== system PMSM_MPCC/MPCC/Subsystem5 ==
  iq_k : Inport
  id_k : Inport  Port=2
  we : Inport  Port=3
  theta_2pi : Inport  Port=4
  Iq_ref : Inport  Port=5
  Id_ref : Inport  Port=6
  Ua : Inport  Port=7
  Ub : Inport  Port=8
  Uc : Inport  Port=9
  Abs : Abs  SaturateOnIntegerOverflow=off
  Abs1 : Abs  SaturateOnIntegerOverflow=off
  Add : Sum
  Clark_Conv1 : Subsystem
  Delay : Delay  Commented=through  DelayLength=1
  Delay1 : Delay  Commented=through  DelayLength=1
  Gain1 : Gain  Gain=Vdc
  Gain2 : Gain  Gain=Vdc
  Gain3 : Gain  Gain=Vdc
  Ls : Constant  Value=Ls
  MATLAB Function : MATLAB Function  TreatAsAtomicUnit=on
  MATLAB Function1 : MATLAB Function  TreatAsAtomicUnit=on
  Memory1 : Memory
  Memory2 : Memory
  Park_Conv1 : Subsystem
  Rs : Constant  Value=Rs
  Sum : Sum  Inputs=|+-
  Sum1 : Sum  Inputs=|+-
  Ts : Constant  Value=1/F
  Ts3 : Constant  Value=psi_f
  J : Outport
  wires:
  Uc/1 -> Gain3/1
  Ub/1 -> Gain2/1
  iq_k/1 -> MATLAB Function/6(iq_k)
  id_k/1 -> MATLAB Function/5(id_k)
  Clark_Conv1/1(Ualpha) -> Park_Conv1/2(Ualpha)
  Abs1/1 -> Add/2
  Ts3/1 -> MATLAB Function/9(psi_f), MATLAB Function1/9(psi_f)
  Ua/1 -> Gain1/1
  Delay1/1 -> Memory2/1
  we/1 -> MATLAB Function1/4(we), MATLAB Function/4(we)
  Id_ref/1 -> Sum/1
  Abs/1 -> Add/1
  Gain3/1 -> Clark_Conv1/3(Uc)
  Sum1/1 -> Abs1/1
  Clark_Conv1/2(Ubeta) -> Park_Conv1/3(Ubeta)
  Ls/1 -> MATLAB Function/3(Ls), MATLAB Function1/3(Ls)
  Gain2/1 -> Clark_Conv1/2(Ub)
  Gain1/1 -> Clark_Conv1/1(Ua)
  Park_Conv1/2(Ud) -> MATLAB Function/7(ud_k), Delay1/1
  MATLAB Function/1(id_k_1) -> MATLAB Function1/5(id_k_1)
  Ts/1 -> MATLAB Function/1(T), MATLAB Function1/1(T)
  Add/1 -> J/1
  MATLAB Function1/1(id_k_2) -> Sum/2
  Delay/1 -> Memory1/1
  Rs/1 -> MATLAB Function/2(Rs), MATLAB Function1/2(Rs)
  MATLAB Function/2(iq_k_1) -> MATLAB Function1/6(iq_k_1)
  Sum/1 -> Abs/1
  theta_2pi/1 -> Park_Conv1/1(theta_2pi)
  Iq_ref/1 -> Sum1/1
  MATLAB Function1/2(iq_k_2) -> Sum1/2
  Park_Conv1/1(Uq) -> MATLAB Function/8(uq_k), Delay/1
  Memory1/1 -> MATLAB Function1/8(uq_k_1)
  Memory2/1 -> MATLAB Function1/7(ud_k_1)

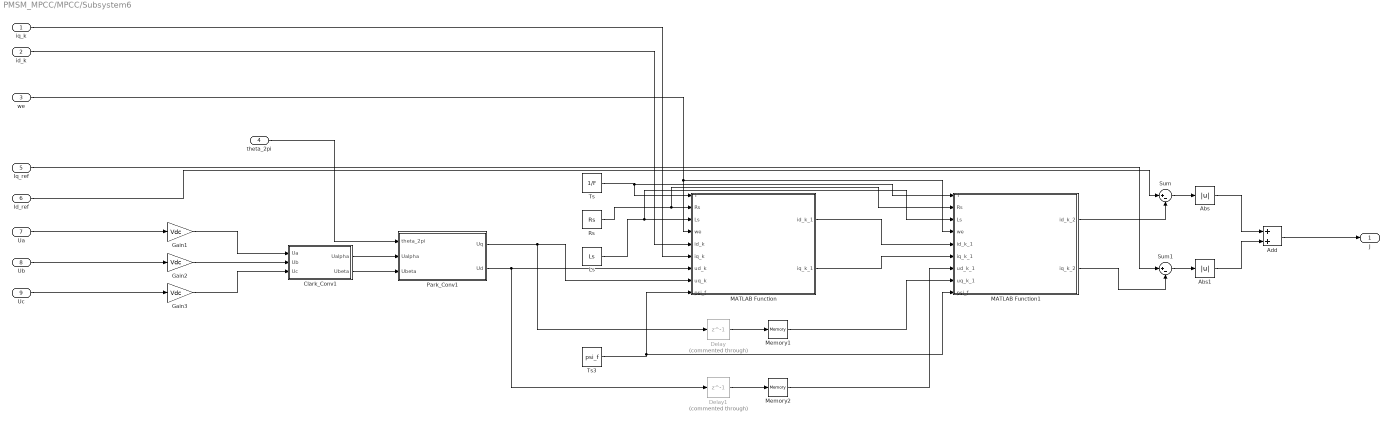
== system PMSM_MPCC/MPCC/Subsystem6 ==
  iq_k : Inport
  id_k : Inport  Port=2
  we : Inport  Port=3
  theta_2pi : Inport  Port=4
  Iq_ref : Inport  Port=5
  Id_ref : Inport  Port=6
  Ua : Inport  Port=7
  Ub : Inport  Port=8
  Uc : Inport  Port=9
  Abs : Abs  SaturateOnIntegerOverflow=off
  Abs1 : Abs  SaturateOnIntegerOverflow=off
  Add : Sum
  Clark_Conv1 : Subsystem
  Delay : Delay  Commented=through  DelayLength=1
  Delay1 : Delay  Commented=through  DelayLength=1
  Gain1 : Gain  Gain=Vdc
  Gain2 : Gain  Gain=Vdc
  Gain3 : Gain  Gain=Vdc
  Ls : Constant  Value=Ls
  MATLAB Function : MATLAB Function  TreatAsAtomicUnit=on
  MATLAB Function1 : MATLAB Function  TreatAsAtomicUnit=on
  Memory1 : Memory
  Memory2 : Memory
  Park_Conv1 : Subsystem
  Rs : Constant  Value=Rs
  Sum : Sum  Inputs=|+-
  Sum1 : Sum  Inputs=|+-
  Ts : Constant  Value=1/F
  Ts3 : Constant  Value=psi_f
  J : Outport
  wires:
  Uc/1 -> Gain3/1
  Ub/1 -> Gain2/1
  iq_k/1 -> MATLAB Function/6(iq_k)
  id_k/1 -> MATLAB Function/5(id_k)
  Clark_Conv1/1(Ualpha) -> Park_Conv1/2(Ualpha)
  Abs1/1 -> Add/2
  Ts3/1 -> MATLAB Function/9(psi_f), MATLAB Function1/9(psi_f)
  Ua/1 -> Gain1/1
  Delay1/1 -> Memory2/1
  we/1 -> MATLAB Function1/4(we), MATLAB Function/4(we)
  Id_ref/1 -> Sum/1
  Abs/1 -> Add/1
  Gain3/1 -> Clark_Conv1/3(Uc)
  Sum1/1 -> Abs1/1
  Clark_Conv1/2(Ubeta) -> Park_Conv1/3(Ubeta)
  Ls/1 -> MATLAB Function/3(Ls), MATLAB Function1/3(Ls)
  Gain2/1 -> Clark_Conv1/2(Ub)
  Gain1/1 -> Clark_Conv1/1(Ua)
  Park_Conv1/2(Ud) -> MATLAB Function/7(ud_k), Delay1/1
  MATLAB Function/1(id_k_1) -> MATLAB Function1/5(id_k_1)
  Ts/1 -> MATLAB Function/1(T), MATLAB Function1/1(T)
  Add/1 -> J/1
  MATLAB Function1/1(id_k_2) -> Sum/2
  Delay/1 -> Memory1/1
  Rs/1 -> MATLAB Function/2(Rs), MATLAB Function1/2(Rs)
  MATLAB Function/2(iq_k_1) -> MATLAB Function1/6(iq_k_1)
  Sum/1 -> Abs/1
  theta_2pi/1 -> Park_Conv1/1(theta_2pi)
  Iq_ref/1 -> Sum1/1
  MATLAB Function1/2(iq_k_2) -> Sum1/2
  Park_Conv1/1(Uq) -> MATLAB Function/8(uq_k), Delay/1
  Memory1/1 -> MATLAB Function1/8(uq_k_1)
  Memory2/1 -> MATLAB Function1/7(ud_k_1)

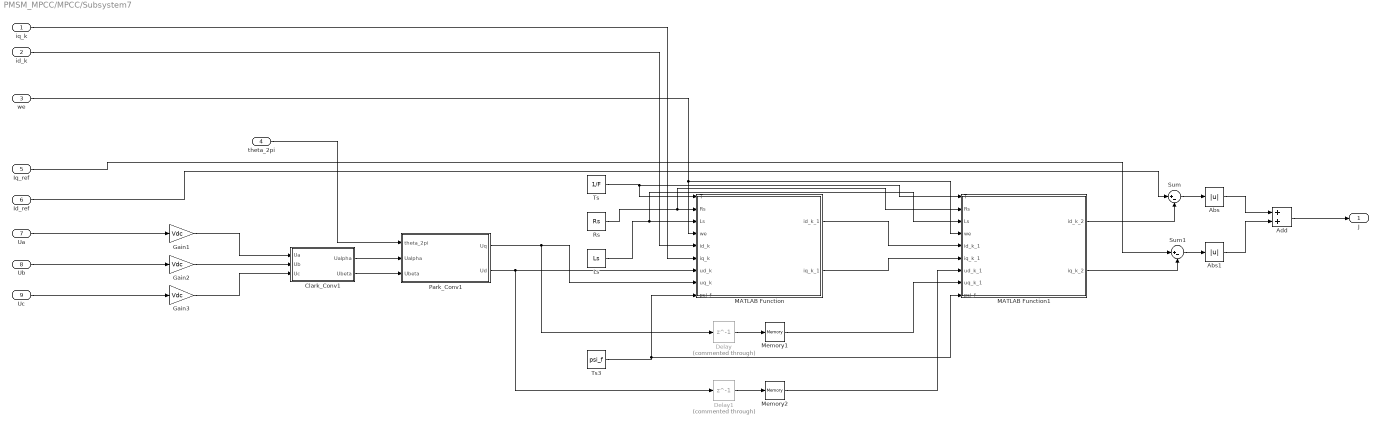
== system PMSM_MPCC/MPCC/Subsystem7 ==
  iq_k : Inport
  id_k : Inport  Port=2
  we : Inport  Port=3
  theta_2pi : Inport  Port=4
  Iq_ref : Inport  Port=5
  Id_ref : Inport  Port=6
  Ua : Inport  Port=7
  Ub : Inport  Port=8
  Uc : Inport  Port=9
  Abs : Abs  SaturateOnIntegerOverflow=off
  Abs1 : Abs  SaturateOnIntegerOverflow=off
  Add : Sum
  Clark_Conv1 : Subsystem
  Delay : Delay  Commented=through  DelayLength=1
  Delay1 : Delay  Commented=through  DelayLength=1
  Gain1 : Gain  Gain=Vdc
  Gain2 : Gain  Gain=Vdc
  Gain3 : Gain  Gain=Vdc
  Ls : Constant  Value=Ls
  MATLAB Function : MATLAB Function  TreatAsAtomicUnit=on
  MATLAB Function1 : MATLAB Function  TreatAsAtomicUnit=on
  Memory1 : Memory
  Memory2 : Memory
  Park_Conv1 : Subsystem
  Rs : Constant  Value=Rs
  Sum : Sum  Inputs=|+-
  Sum1 : Sum  Inputs=|+-
  Ts : Constant  Value=1/F
  Ts3 : Constant  Value=psi_f
  J : Outport
  wires:
  Uc/1 -> Gain3/1
  Ub/1 -> Gain2/1
  iq_k/1 -> MATLAB Function/6(iq_k)
  id_k/1 -> MATLAB Function/5(id_k)
  Clark_Conv1/1(Ualpha) -> Park_Conv1/2(Ualpha)
  Abs1/1 -> Add/2
  Ts3/1 -> MATLAB Function/9(psi_f), MATLAB Function1/9(psi_f)
  Ua/1 -> Gain1/1
  Delay1/1 -> Memory2/1
  we/1 -> MATLAB Function1/4(we), MATLAB Function/4(we)
  Id_ref/1 -> Sum/1
  Abs/1 -> Add/1
  Gain3/1 -> Clark_Conv1/3(Uc)
  Sum1/1 -> Abs1/1
  Clark_Conv1/2(Ubeta) -> Park_Conv1/3(Ubeta)
  Ls/1 -> MATLAB Function/3(Ls), MATLAB Function1/3(Ls)
  Gain2/1 -> Clark_Conv1/2(Ub)
  Gain1/1 -> Clark_Conv1/1(Ua)
  Park_Conv1/2(Ud) -> MATLAB Function/7(ud_k), Delay1/1
  MATLAB Function/1(id_k_1) -> MATLAB Function1/5(id_k_1)
  Ts/1 -> MATLAB Function/1(T), MATLAB Function1/1(T)
  Add/1 -> J/1
  MATLAB Function1/1(id_k_2) -> Sum/2
  Delay/1 -> Memory1/1
  Rs/1 -> MATLAB Function/2(Rs), MATLAB Function1/2(Rs)
  MATLAB Function/2(iq_k_1) -> MATLAB Function1/6(iq_k_1)
  Sum/1 -> Abs/1
  theta_2pi/1 -> Park_Conv1/1(theta_2pi)
  Iq_ref/1 -> Sum1/1
  MATLAB Function1/2(iq_k_2) -> Sum1/2
  Park_Conv1/1(Uq) -> MATLAB Function/8(uq_k), Delay/1
  Memory1/1 -> MATLAB Function1/8(uq_k_1)
  Memory2/1 -> MATLAB Function1/7(ud_k_1)

== system PMSM_MPCC/Filter/LowpassFilter/Lowpass filter1 ==
  K : Inport
  u(t) : Inport  Port=2
  Add : Sum
  Delay : Delay  DelayLength=1
  Product : Product
  Subtract : Sum  Inputs=+-
  Ia : Outport
  wires:
  Add/1 -> Ia/1, Delay/1
  Product/1 -> Add/1
  Subtract/1 -> Product/2
  Delay/1 -> Subtract/2, Add/2
  K/1 -> Product/1
  u(t)/1 -> Subtract/1

== system PMSM_MPCC/Filter/LowpassFilter/Lowpass filter2 ==
  K : Inport
  u(t) : Inport  Port=2
  Add : Sum
  Delay : Delay  DelayLength=1
  Product : Product
  Subtract : Sum  Inputs=+-
  Ib : Outport
  wires:
  u(t)/1 -> Subtract/1
  K/1 -> Product/1
  Delay/1 -> Add/2, Subtract/2
  Subtract/1 -> Product/2
  Product/1 -> Add/1
  Add/1 -> Delay/1, Ib/1

== system PMSM_MPCC/Filter/LowpassFilter/Lowpass filter3 ==
  K : Inport
  u(t) : Inport  Port=2
  Add : Sum
  Delay : Delay  DelayLength=1
  Product : Product
  Subtract : Sum  Inputs=+-
  Ic : Outport
  wires:
  Add/1 -> Ic/1, Delay/1
  Product/1 -> Add/1
  Subtract/1 -> Product/2
  Delay/1 -> Subtract/2, Add/2
  K/1 -> Product/1
  u(t)/1 -> Subtract/1

== system PMSM_MPCC/MPCC/Subsystem/Clark_Conv1 ==
  Ua : Inport
  Ub : Inport  Port=2
  Uc : Inport  Port=3
  Add : Sum  Inputs=+-  OutDataTypeStr=double
  Gain : Gain  Gain=sqrt(3)  ParamDataTypeStr=double
  Gain2 : Gain  Gain=0.5
  Gain3 : Gain  Gain=0.5
  Subtract : Sum  Inputs=+--  OutDataTypeStr=double
  Ualpha : Outport
  Ubeta : Outport  Port=2
  wires:
  Ua/1 -> Subtract/1
  Ub/1 -> Gain2/1
  Add/1 -> Gain/1
  Gain/1 -> Ubeta/1
  Uc/1 -> Gain3/1
  Gain2/1 -> Subtract/2, Add/1
  Gain3/1 -> Subtract/3, Add/2
  Subtract/1 -> Ualpha/1

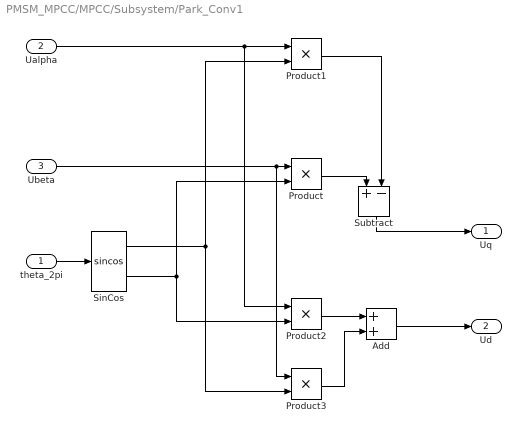
== system PMSM_MPCC/MPCC/Subsystem/Park_Conv1 ==
  theta_2pi : Inport
  Ualpha : Inport  Port=2
  Ubeta : Inport  Port=3
  Add : Sum
  Product{,1..3} (4 alike) : Product
  SinCos : Trigonometry  Operator=sincos
  Subtract : Sum  Inputs=+-
  Uq : Outport
  Ud : Outport  Port=2
  wires:
  Ualpha/1 -> Product1/1, Product2/1
  Ubeta/1 -> Product3/1, Product/1
  theta_2pi/1 -> SinCos/1
  SinCos/2 -> Product2/2, Product/2
  SinCos/1 -> Product3/2, Product1/2
  Product1/1 -> Subtract/2
  Subtract/1 -> Uq/1
  Product/1 -> Subtract/1
  Product2/1 -> Add/1
  Product3/1 -> Add/2
  Add/1 -> Ud/1

== system PMSM_MPCC/MPCC/Subsystem1/Clark_Conv1 ==
  Ua : Inport
  Ub : Inport  Port=2
  Uc : Inport  Port=3
  Add : Sum  Inputs=+-  OutDataTypeStr=double
  Gain : Gain  Gain=sqrt(3)  ParamDataTypeStr=double
  Gain2 : Gain  Gain=0.5
  Gain3 : Gain  Gain=0.5
  Subtract : Sum  Inputs=+--  OutDataTypeStr=double
  Ualpha : Outport
  Ubeta : Outport  Port=2
  wires:
  Subtract/1 -> Ualpha/1
  Gain3/1 -> Add/2, Subtract/3
  Gain2/1 -> Add/1, Subtract/2
  Uc/1 -> Gain3/1
  Gain/1 -> Ubeta/1
  Add/1 -> Gain/1
  Ub/1 -> Gain2/1
  Ua/1 -> Subtract/1

== system PMSM_MPCC/MPCC/Subsystem1/Park_Conv1 ==
  theta_2pi : Inport
  Ualpha : Inport  Port=2
  Ubeta : Inport  Port=3
  Add : Sum
  Product{,1..3} (4 alike) : Product
  SinCos : Trigonometry  Operator=sincos
  Subtract : Sum  Inputs=+-
  Uq : Outport
  Ud : Outport  Port=2
  wires:
  Add/1 -> Ud/1
  Product3/1 -> Add/2
  Product2/1 -> Add/1
  Product/1 -> Subtract/1
  Subtract/1 -> Uq/1
  Product1/1 -> Subtract/2
  SinCos/1 -> Product1/2, Product3/2
  SinCos/2 -> Product/2, Product2/2
  theta_2pi/1 -> SinCos/1
  Ubeta/1 -> Product/1, Product3/1
  Ualpha/1 -> Product2/1, Product1/1

== system PMSM_MPCC/MPCC/Subsystem2/Clark_Conv1 ==
  Ua : Inport
  Ub : Inport  Port=2
  Uc : Inport  Port=3
  Add : Sum  Inputs=+-  OutDataTypeStr=double
  Gain : Gain  Gain=sqrt(3)  ParamDataTypeStr=double
  Gain2 : Gain  Gain=0.5
  Gain3 : Gain  Gain=0.5
  Subtract : Sum  Inputs=+--  OutDataTypeStr=double
  Ualpha : Outport
  Ubeta : Outport  Port=2
  wires:
  Subtract/1 -> Ualpha/1
  Gain3/1 -> Add/2, Subtract/3
  Gain2/1 -> Add/1, Subtract/2
  Uc/1 -> Gain3/1
  Gain/1 -> Ubeta/1
  Add/1 -> Gain/1
  Ub/1 -> Gain2/1
  Ua/1 -> Subtract/1

== system PMSM_MPCC/MPCC/Subsystem2/Park_Conv1 ==
  theta_2pi : Inport
  Ualpha : Inport  Port=2
  Ubeta : Inport  Port=3
  Add : Sum
  Product{,1..3} (4 alike) : Product
  SinCos : Trigonometry  Operator=sincos
  Subtract : Sum  Inputs=+-
  Uq : Outport
  Ud : Outport  Port=2
  wires:
  Add/1 -> Ud/1
  Product3/1 -> Add/2
  Product2/1 -> Add/1
  Product/1 -> Subtract/1
  Subtract/1 -> Uq/1
  Product1/1 -> Subtract/2
  SinCos/1 -> Product1/2, Product3/2
  SinCos/2 -> Product/2, Product2/2
  theta_2pi/1 -> SinCos/1
  Ubeta/1 -> Product/1, Product3/1
  Ualpha/1 -> Product2/1, Product1/1

== system PMSM_MPCC/MPCC/Subsystem3/Clark_Conv1 ==
  Ua : Inport
  Ub : Inport  Port=2
  Uc : Inport  Port=3
  Add : Sum  Inputs=+-  OutDataTypeStr=double
  Gain : Gain  Gain=sqrt(3)  ParamDataTypeStr=double
  Gain2 : Gain  Gain=0.5
  Gain3 : Gain  Gain=0.5
  Subtract : Sum  Inputs=+--  OutDataTypeStr=double
  Ualpha : Outport
  Ubeta : Outport  Port=2
  wires:
  Subtract/1 -> Ualpha/1
  Gain3/1 -> Add/2, Subtract/3
  Gain2/1 -> Add/1, Subtract/2
  Uc/1 -> Gain3/1
  Gain/1 -> Ubeta/1
  Add/1 -> Gain/1
  Ub/1 -> Gain2/1
  Ua/1 -> Subtract/1

== system PMSM_MPCC/MPCC/Subsystem3/Park_Conv1 ==
  theta_2pi : Inport
  Ualpha : Inport  Port=2
  Ubeta : Inport  Port=3
  Add : Sum
  Product{,1..3} (4 alike) : Product
  SinCos : Trigonometry  Operator=sincos
  Subtract : Sum  Inputs=+-
  Uq : Outport
  Ud : Outport  Port=2
  wires:
  Add/1 -> Ud/1
  Product3/1 -> Add/2
  Product2/1 -> Add/1
  Product/1 -> Subtract/1
  Subtract/1 -> Uq/1
  Product1/1 -> Subtract/2
  SinCos/1 -> Product1/2, Product3/2
  SinCos/2 -> Product/2, Product2/2
  theta_2pi/1 -> SinCos/1
  Ubeta/1 -> Product/1, Product3/1
  Ualpha/1 -> Product2/1, Product1/1

== system PMSM_MPCC/MPCC/Subsystem4/Clark_Conv1 ==
  Ua : Inport
  Ub : Inport  Port=2
  Uc : Inport  Port=3
  Add : Sum  Inputs=+-  OutDataTypeStr=double
  Gain : Gain  Gain=sqrt(3)  ParamDataTypeStr=double
  Gain2 : Gain  Gain=0.5
  Gain3 : Gain  Gain=0.5
  Subtract : Sum  Inputs=+--  OutDataTypeStr=double
  Ualpha : Outport
  Ubeta : Outport  Port=2
  wires:
  Subtract/1 -> Ualpha/1
  Gain3/1 -> Add/2, Subtract/3
  Gain2/1 -> Add/1, Subtract/2
  Uc/1 -> Gain3/1
  Gain/1 -> Ubeta/1
  Add/1 -> Gain/1
  Ub/1 -> Gain2/1
  Ua/1 -> Subtract/1

== system PMSM_MPCC/MPCC/Subsystem4/Park_Conv1 ==
  theta_2pi : Inport
  Ualpha : Inport  Port=2
  Ubeta : Inport  Port=3
  Add : Sum
  Product{,1..3} (4 alike) : Product
  SinCos : Trigonometry  Operator=sincos
  Subtract : Sum  Inputs=+-
  Uq : Outport
  Ud : Outport  Port=2
  wires:
  Add/1 -> Ud/1
  Product3/1 -> Add/2
  Product2/1 -> Add/1
  Product/1 -> Subtract/1
  Subtract/1 -> Uq/1
  Product1/1 -> Subtract/2
  SinCos/1 -> Product1/2, Product3/2
  SinCos/2 -> Product/2, Product2/2
  theta_2pi/1 -> SinCos/1
  Ubeta/1 -> Product/1, Product3/1
  Ualpha/1 -> Product2/1, Product1/1

== system PMSM_MPCC/MPCC/Subsystem5/Clark_Conv1 ==
  Ua : Inport
  Ub : Inport  Port=2
  Uc : Inport  Port=3
  Add : Sum  Inputs=+-  OutDataTypeStr=double
  Gain : Gain  Gain=sqrt(3)  ParamDataTypeStr=double
  Gain2 : Gain  Gain=0.5
  Gain3 : Gain  Gain=0.5
  Subtract : Sum  Inputs=+--  OutDataTypeStr=double
  Ualpha : Outport
  Ubeta : Outport  Port=2
  wires:
  Subtract/1 -> Ualpha/1
  Gain3/1 -> Add/2, Subtract/3
  Gain2/1 -> Add/1, Subtract/2
  Uc/1 -> Gain3/1
  Gain/1 -> Ubeta/1
  Add/1 -> Gain/1
  Ub/1 -> Gain2/1
  Ua/1 -> Subtract/1

== system PMSM_MPCC/MPCC/Subsystem5/Park_Conv1 ==
  theta_2pi : Inport
  Ualpha : Inport  Port=2
  Ubeta : Inport  Port=3
  Add : Sum
  Product{,1..3} (4 alike) : Product
  SinCos : Trigonometry  Operator=sincos
  Subtract : Sum  Inputs=+-
  Uq : Outport
  Ud : Outport  Port=2
  wires:
  Add/1 -> Ud/1
  Product3/1 -> Add/2
  Product2/1 -> Add/1
  Product/1 -> Subtract/1
  Subtract/1 -> Uq/1
  Product1/1 -> Subtract/2
  SinCos/1 -> Product1/2, Product3/2
  SinCos/2 -> Product/2, Product2/2
  theta_2pi/1 -> SinCos/1
  Ubeta/1 -> Product/1, Product3/1
  Ualpha/1 -> Product2/1, Product1/1

== system PMSM_MPCC/MPCC/Subsystem6/Clark_Conv1 ==
  Ua : Inport
  Ub : Inport  Port=2
  Uc : Inport  Port=3
  Add : Sum  Inputs=+-  OutDataTypeStr=double
  Gain : Gain  Gain=sqrt(3)  ParamDataTypeStr=double
  Gain2 : Gain  Gain=0.5
  Gain3 : Gain  Gain=0.5
  Subtract : Sum  Inputs=+--  OutDataTypeStr=double
  Ualpha : Outport
  Ubeta : Outport  Port=2
  wires:
  Subtract/1 -> Ualpha/1
  Gain3/1 -> Add/2, Subtract/3
  Gain2/1 -> Add/1, Subtract/2
  Uc/1 -> Gain3/1
  Gain/1 -> Ubeta/1
  Add/1 -> Gain/1
  Ub/1 -> Gain2/1
  Ua/1 -> Subtract/1

== system PMSM_MPCC/MPCC/Subsystem6/Park_Conv1 ==
  theta_2pi : Inport
  Ualpha : Inport  Port=2
  Ubeta : Inport  Port=3
  Add : Sum
  Product{,1..3} (4 alike) : Product
  SinCos : Trigonometry  Operator=sincos
  Subtract : Sum  Inputs=+-
  Uq : Outport
  Ud : Outport  Port=2
  wires:
  Add/1 -> Ud/1
  Product3/1 -> Add/2
  Product2/1 -> Add/1
  Product/1 -> Subtract/1
  Subtract/1 -> Uq/1
  Product1/1 -> Subtract/2
  SinCos/1 -> Product1/2, Product3/2
  SinCos/2 -> Product/2, Product2/2
  theta_2pi/1 -> SinCos/1
  Ubeta/1 -> Product/1, Product3/1
  Ualpha/1 -> Product2/1, Product1/1

== system PMSM_MPCC/MPCC/Subsystem7/Clark_Conv1 ==
  Ua : Inport
  Ub : Inport  Port=2
  Uc : Inport  Port=3
  Add : Sum  Inputs=+-  OutDataTypeStr=double
  Gain : Gain  Gain=sqrt(3)  ParamDataTypeStr=double
  Gain2 : Gain  Gain=0.5
  Gain3 : Gain  Gain=0.5
  Subtract : Sum  Inputs=+--  OutDataTypeStr=double
  Ualpha : Outport
  Ubeta : Outport  Port=2
  wires:
  Subtract/1 -> Ualpha/1
  Gain3/1 -> Add/2, Subtract/3
  Gain2/1 -> Add/1, Subtract/2
  Uc/1 -> Gain3/1
  Gain/1 -> Ubeta/1
  Add/1 -> Gain/1
  Ub/1 -> Gain2/1
  Ua/1 -> Subtract/1

== system PMSM_MPCC/MPCC/Subsystem7/Park_Conv1 ==
  theta_2pi : Inport
  Ualpha : Inport  Port=2
  Ubeta : Inport  Port=3
  Add : Sum
  Product{,1..3} (4 alike) : Product
  SinCos : Trigonometry  Operator=sincos
  Subtract : Sum  Inputs=+-
  Uq : Outport
  Ud : Outport  Port=2
  wires:
  Add/1 -> Ud/1
  Product3/1 -> Add/2
  Product2/1 -> Add/1
  Product/1 -> Subtract/1
  Subtract/1 -> Uq/1
  Product1/1 -> Subtract/2
  SinCos/1 -> Product1/2, Product3/2
  SinCos/2 -> Product/2, Product2/2
  theta_2pi/1 -> SinCos/1
  Ubeta/1 -> Product/1, Product3/1
  Ualpha/1 -> Product2/1, Product1/1

== matlab function PMSM_MPCC/MPCC/Subsystem2/MATLAB Function1 ==
  data: T input; id_k_2 output; Rs input; Ls input; we input; id_k_1 input; iq_k_1 input; ud_k_1 input; uq_k_1 input; iq_k_2 output; psi_f input
function [id_k_2,iq_k_2] = fcn(T,Rs,Ls,we,id_k_1,iq_k_1,ud_k_1,uq_k_1,psi_f)

id_k_2 = (1-T*Rs/Ls)*id_k_1+T/Ls*ud_k_1+T*we*iq_k_1;
iq_k_2 = (1-T*Rs/Ls)*iq_k_1+T/Ls*uq_k_1-T*we*id_k_1-T*we*psi_f/Ls;

== matlab function PMSM_MPCC/MPCC/Subsystem3/MATLAB Function ==
  data: T input; id_k_1 output; Rs input; Ls input; we input; id_k input; iq_k input; ud_k input; uq_k input; iq_k_1 output; psi_f input
function [id_k_1,iq_k_1] = fcn(T,Rs,Ls,we,id_k,iq_k,ud_k,uq_k,psi_f)

id_k_1 = (1-T*Rs/Ls)*id_k+T/Ls*ud_k+T*we*iq_k;
iq_k_1 = (1-T*Rs/Ls)*iq_k+T/Ls*uq_k-T*we*id_k-T*we*psi_f/Ls;

== matlab function PMSM_MPCC/MPCC/Subsystem3/MATLAB Function1 ==
  data: T input; id_k_2 output; Rs input; Ls input; we input; id_k_1 input; iq_k_1 input; ud_k_1 input; uq_k_1 input; iq_k_2 output; psi_f input
function [id_k_2,iq_k_2] = fcn(T,Rs,Ls,we,id_k_1,iq_k_1,ud_k_1,uq_k_1,psi_f)

id_k_2 = (1-T*Rs/Ls)*id_k_1+T/Ls*ud_k_1+T*we*iq_k_1;
iq_k_2 = (1-T*Rs/Ls)*iq_k_1+T/Ls*uq_k_1-T*we*id_k_1-T*we*psi_f/Ls;

== matlab function PMSM_MPCC/MPCC/Subsystem4/MATLAB Function ==
  data: T input; id_k_1 output; Rs input; Ls input; we input; id_k input; iq_k input; ud_k input; uq_k input; iq_k_1 output; psi_f input
function [id_k_1,iq_k_1] = fcn(T,Rs,Ls,we,id_k,iq_k,ud_k,uq_k,psi_f)

id_k_1 = (1-T*Rs/Ls)*id_k+T/Ls*ud_k+T*we*iq_k;
iq_k_1 = (1-T*Rs/Ls)*iq_k+T/Ls*uq_k-T*we*id_k-T*we*psi_f/Ls;

== matlab function PMSM_MPCC/MATLAB Function ==
  data: angle input; theta_2pi output
function theta_2pi = Angle_Conv(angle)

theta_2pi=mod(angle,2*pi);

== matlab function PMSM_MPCC/MPCC/Subsystem4/MATLAB Function1 ==
  data: T input; id_k_2 output; Rs input; Ls input; we input; id_k_1 input; iq_k_1 input; ud_k_1 input; uq_k_1 input; iq_k_2 output; psi_f input
function [id_k_2,iq_k_2] = fcn(T,Rs,Ls,we,id_k_1,iq_k_1,ud_k_1,uq_k_1,psi_f)

id_k_2 = (1-T*Rs/Ls)*id_k_1+T/Ls*ud_k_1+T*we*iq_k_1;
iq_k_2 = (1-T*Rs/Ls)*iq_k_1+T/Ls*uq_k_1-T*we*id_k_1-T*we*psi_f/Ls;

== matlab function PMSM_MPCC/MPCC/Subsystem5/MATLAB Function ==
  data: T input; id_k_1 output; Rs input; Ls input; we input; id_k input; iq_k input; ud_k input; uq_k input; iq_k_1 output; psi_f input
function [id_k_1,iq_k_1] = fcn(T,Rs,Ls,we,id_k,iq_k,ud_k,uq_k,psi_f)

id_k_1 = (1-T*Rs/Ls)*id_k+T/Ls*ud_k+T*we*iq_k;
iq_k_1 = (1-T*Rs/Ls)*iq_k+T/Ls*uq_k-T*we*id_k-T*we*psi_f/Ls;

== matlab function PMSM_MPCC/MPCC/Subsystem5/MATLAB Function1 ==
  data: T input; id_k_2 output; Rs input; Ls input; we input; id_k_1 input; iq_k_1 input; ud_k_1 input; uq_k_1 input; iq_k_2 output; psi_f input
function [id_k_2,iq_k_2] = fcn(T,Rs,Ls,we,id_k_1,iq_k_1,ud_k_1,uq_k_1,psi_f)

id_k_2 = (1-T*Rs/Ls)*id_k_1+T/Ls*ud_k_1+T*we*iq_k_1;
iq_k_2 = (1-T*Rs/Ls)*iq_k_1+T/Ls*uq_k_1-T*we*id_k_1-T*we*psi_f/Ls;

== matlab function PMSM_MPCC/MPCC/Subsystem6/MATLAB Function ==
  data: T input; id_k_1 output; Rs input; Ls input; we input; id_k input; iq_k input; ud_k input; uq_k input; iq_k_1 output; psi_f input
function [id_k_1,iq_k_1] = fcn(T,Rs,Ls,we,id_k,iq_k,ud_k,uq_k,psi_f)

id_k_1 = (1-T*Rs/Ls)*id_k+T/Ls*ud_k+T*we*iq_k;
iq_k_1 = (1-T*Rs/Ls)*iq_k+T/Ls*uq_k-T*we*id_k-T*we*psi_f/Ls;

== matlab function PMSM_MPCC/MPCC/Subsystem/一拍延时补偿电流 ==
  data: T input; id_k_1 output; Rs input; Ls input; we input; id_k input; iq_k input; ud_k input; uq_k input; iq_k_1 output; psi_f input
function [id_k_1,iq_k_1] = fcn(T,Rs,Ls,we,id_k,iq_k,ud_k,uq_k,psi_f)

id_k_1 = (1-T*Rs/Ls)*id_k+T/Ls*ud_k+T*we*iq_k;
iq_k_1 = (1-T*Rs/Ls)*iq_k+T/Ls*uq_k-T*we*id_k-T*we*psi_f/Ls;

== matlab function PMSM_MPCC/MPCC/Subsystem6/MATLAB Function1 ==
  data: T input; id_k_2 output; Rs input; Ls input; we input; id_k_1 input; iq_k_1 input; ud_k_1 input; uq_k_1 input; iq_k_2 output; psi_f input
function [id_k_2,iq_k_2] = fcn(T,Rs,Ls,we,id_k_1,iq_k_1,ud_k_1,uq_k_1,psi_f)

id_k_2 = (1-T*Rs/Ls)*id_k_1+T/Ls*ud_k_1+T*we*iq_k_1;
iq_k_2 = (1-T*Rs/Ls)*iq_k_1+T/Ls*uq_k_1-T*we*id_k_1-T*we*psi_f/Ls;

== matlab function PMSM_MPCC/MPCC/Subsystem7/MATLAB Function ==
  data: T input; id_k_1 output; Rs input; Ls input; we input; id_k input; iq_k input; ud_k input; uq_k input; iq_k_1 output; psi_f input
function [id_k_1,iq_k_1] = fcn(T,Rs,Ls,we,id_k,iq_k,ud_k,uq_k,psi_f)

id_k_1 = (1-T*Rs/Ls)*id_k+T/Ls*ud_k+T*we*iq_k;
iq_k_1 = (1-T*Rs/Ls)*iq_k+T/Ls*uq_k-T*we*id_k-T*we*psi_f/Ls;

== matlab function PMSM_MPCC/MPCC/Subsystem7/MATLAB Function1 ==
  data: T input; id_k_2 output; Rs input; Ls input; we input; id_k_1 input; iq_k_1 input; ud_k_1 input; uq_k_1 input; iq_k_2 output; psi_f input
function [id_k_2,iq_k_2] = fcn(T,Rs,Ls,we,id_k_1,iq_k_1,ud_k_1,uq_k_1,psi_f)

id_k_2 = (1-T*Rs/Ls)*id_k_1+T/Ls*ud_k_1+T*we*iq_k_1;
iq_k_2 = (1-T*Rs/Ls)*iq_k_1+T/Ls*uq_k_1-T*we*id_k_1-T*we*psi_f/Ls;
